simulink subsystem "ALU_1bit_SS"  (R2022a)
settings: Solver=VariableStepAuto  StartTime=0.0  StopTime=10.0  RelTol=1e-3
libraries: hdlBasic x8
settings Model: Creator=viktor  LastModifiedBy=viktor

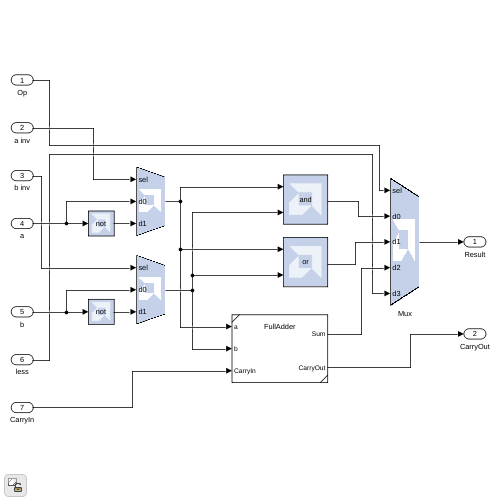
[thumbnail: Simulink's stored preview of the top-level diagram]
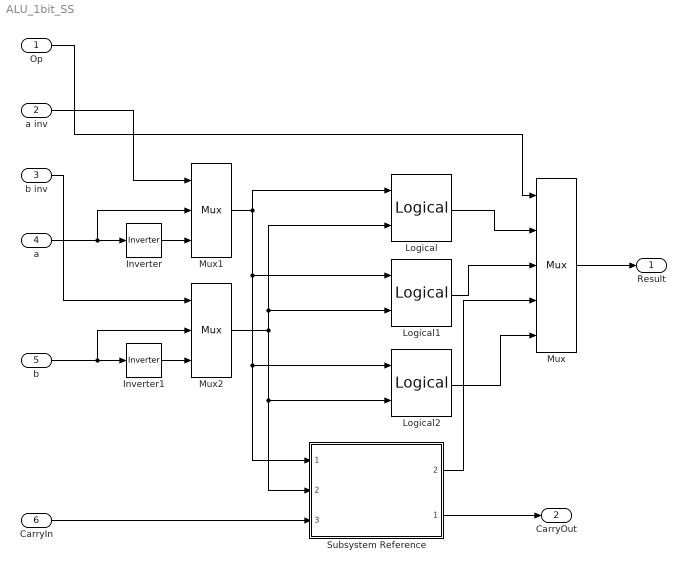
== system ALU_1bit_SS ==
  Op : Inport
  a inv : Inport  Port=2
  b inv : Inport  Port=3
  a : Inport  Port=4
  b : Inport  Port=5
  CarryIn : Inport  Port=6
  Inverter : hdlBasic/Inverter  en=off  latency=0  XmcBlockStatus=1  maskContainerNames=group2  block_type=inv  block_config=sysgen:Inverter_config
  Inverter1 : hdlBasic/Inverter  en=off  latency=0  XmcBlockStatus=1  maskContainerNames=group2  block_type=inv  block_config=sysgen:Inverter_config
  Logical : hdlBasic/Logical  logical_function=AND  inputs=2  en=off  latency=0  precision=Full  arith_type=Boolean  n_bits=16  bin_pt=0  align_bp=on  overflow=[]  quantization=[]  XmcBlockStatus=1  maskContainerNames=tabcontainer1  block_type=logical  block_config=sysgen:Logical_config
  Logical1 : hdlBasic/Logical  logical_function=OR  inputs=2  en=off  latency=0  precision=Full  arith_type=Boolean  n_bits=16  bin_pt=0  align_bp=on  overflow=[]  quantization=[]  XmcBlockStatus=1  maskContainerNames=tabcontainer1  block_type=logical  block_config=sysgen:Logical_config
  Logical2 : hdlBasic/Logical  logical_function=XOR  inputs=2  en=off  latency=0  precision=Full  arith_type=Boolean  n_bits=16  bin_pt=0  align_bp=on  overflow=[]  quantization=[]  XmcBlockStatus=1  maskContainerNames=tabcontainer1  block_type=logical  block_config=sysgen:Logical_config
  Mux : hdlBasic/Mux  inputs=4  en=off  latency=0  precision=User Defined  arith_type=Unsigned  n_bits=1  bin_pt=0  quantization=Truncate  overflow=Wrap  XmcBlockStatus=1  maskContainerNames=tabcontainer1  block_type=mux  block_config=sysgen:Mux_config
  Mux1 : hdlBasic/Mux  inputs=2  en=off  latency=0  precision=Full  arith_type=Unsigned  n_bits=16  bin_pt=14  quantization=Truncate  overflow=Wrap  XmcBlockStatus=1  maskContainerNames=tabcontainer1  block_type=mux  block_config=sysgen:Mux_config
  Mux2 : hdlBasic/Mux  inputs=2  en=off  latency=0  precision=Full  arith_type=Unsigned  n_bits=16  bin_pt=14  quantization=Truncate  overflow=Wrap  XmcBlockStatus=1  maskContainerNames=tabcontainer1  block_type=mux  block_config=sysgen:Mux_config
  Subsystem Reference : Subsystem  ReferencedSubsystem=FullAdder
      settings: PortSchema="{\"entries\":[{\"content\":{\"sides\":[{\"content\":{\"connectorIds\":[\"In1\",\"In2\",\"In3\"]},\"type\":\"ConnectorPlacement.EquallySpacedRectSide\",\"uuid\":\"cd64a273-ec86-4986-bddb-c0a9b5444a31\"},{\"content\":{\"connectorIds\":[\"Out2\",\"Out1\"],\"side\":\"RIGHT\"},\"type\":\"ConnectorPlacement.EquallySpacedRectSide\",\"uuid\":\"3856e352-4c74-47c7-995c-212bed1abb9b\"},{\"content\":{\"connectorIds\":[],\"side\":\"TOP\"},\"type\":\"ConnectorPlacement.EquallySpacedRectSide\",\"uuid\":\"2ecd0bf4-056f-4d62-834c-e3d284e44597\"}]},\"type\":\"ConnectorPlacement.EquallySpacedConnector\",\"uuid\":\"444ea574-66b1-4a18-82e3-f1ce24df8662\"}],\"packageUris\":[\"http://schema.mathworks.com/mf0/Connector/R2020b\"],\"version\":\"1.0\"}"
  Result : Outport
  CarryOut : Outport  Port=2
  wires:
  Inverter1/1 -> Mux2/3
  Logical1/1 -> Mux/3
  Mux/1 -> Result/1
  a inv/1 -> Mux1/1
  b inv/1 -> Mux2/1
  Op/1 -> Mux/1
  a/1 -> Inverter/1, Mux1/2
  Mux2/1 -> Logical/2, Logical1/2, Logical2/2, Subsystem Reference/2
  Mux1/1 -> Logical1/1, Subsystem Reference/1, Logical2/1, Logical/1
  b/1 -> Inverter1/1, Mux2/2
  Subsystem Reference/2 -> Mux/4
  CarryIn/1 -> Subsystem Reference/3
  Inverter/1 -> Mux1/3
  Logical/1 -> Mux/2
  Subsystem Reference/1 -> CarryOut/1
  Logical2/1 -> Mux/5
